simulink library "libFSArray"  (R2020a)
settings: Solver=VariableStepAuto  StartTime=0.0  StopTime=10.0  RelTol=1e-3
libraries: powerlib x2, $bdroot x1, re_lib x1
settings Model: Creator=pkoralew  LastModifiedBy=pkoralew

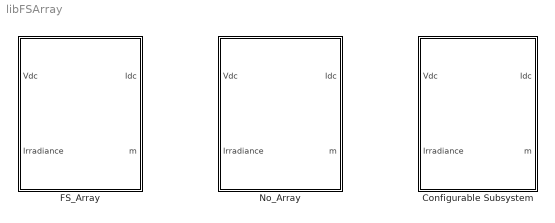
== system libFSArray ==
  Configurable Subsystem : Subsystem  BlockChoice=FS_Array
      settings: TemplateBlock=self  MemberBlocks=FS_Array,No_Array
  FS_Array : Subsystem
  No_Array : Subsystem

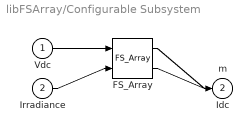
== system libFSArray/Configurable Subsystem ==
  Vdc : Inport
  Irradiance : Inport  Port=2
  FS_Array : $bdroot/FS_Array  SystemSampleTime=-1  Latency=0  AutoFrameSizeCalculation=off
  Idc : Outport
  m : Outport  Port=2
  wires:
  Vdc/1 -> FS_Array/1
  Irradiance/1 -> FS_Array/2
  FS_Array/1 -> Idc/1
  FS_Array/2 -> m/1

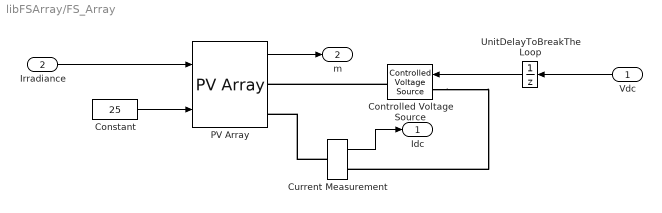
== system libFSArray/FS_Array ==
  Vdc : Inport
  Irradiance : Inport  Port=2
  Constant : Constant  Value=25
  Controlled Voltage Source : powerlib/Electrical Sources/Controlled Voltage Source  Initialize=on  Source_Type=AC  Amplitude=0  Phase=0  Frequency=0  Measurements=None
  Current Measurement : powerlib/Measurements/Current Measurement  PhasorSimulation=off  OutputType=Complex  PSBequivalent=0
  PV Array : re_lib/Solar/PV Array  Npar=300  Nser=18  PlotType=array @ 1000 W/m2 & specified temperatures  S_vec="[ 1000  500  100 ]"  Temp_C_vec="[ 45 25  ]"  ModuleName=First Solar FS-390  PlotWhenSelected=off  Pm=90.036  Ncell=77  Voc=61  Isc=2.04  Vm=49.2  Im=1.83  beta_Voc_pc=-0.236  alpha_Isc_pc=0.04299  beta_Voc=-0.14396  alpha_Isc=0.000877  IL=2.0554  I0=3.4814e-13  nI=1.0515  Rsh=377.2704  Rs=2.8667  RobustModel=off  RobustCellTemperature=25  BAL=on  Tc=1e-6  Tfilter=5e-5
  UnitDelayToBreakTheLoop : UnitDelay  InitialCondition=1000  SampleTime=-1  HasFrameUpgradeWarning=on
  Idc : Outport
  m : Outport  Port=2
  wires:
  Vdc/1 -> UnitDelayToBreakTheLoop/1
  PV Array/1 -> m/1
  UnitDelayToBreakTheLoop/1 -> Controlled Voltage Source/1
  Current Measurement/1 -> Idc/1
  Constant/1 -> PV Array/2
  Irradiance/1 -> PV Array/1
  connections:
  Controlled Voltage Source/RConn1 -- PV Array/RConn1
  Controlled Voltage Source/LConn1 -- Current Measurement/RConn1
  Current Measurement/LConn1 -- PV Array/RConn2

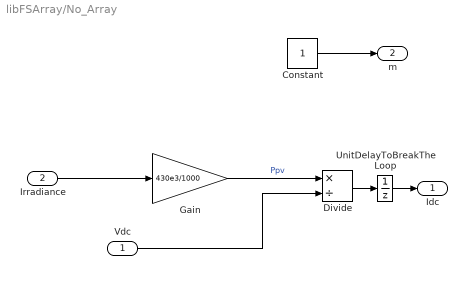
== system libFSArray/No_Array ==
  Vdc : Inport
  Irradiance : Inport  Port=2
  Constant : Constant
  Divide : Product  Inputs=*/
  Gain : Gain  Gain=430e3/1000
  UnitDelayToBreakTheLoop : UnitDelay  InitialCondition=1000  SampleTime=-1  HasFrameUpgradeWarning=on
  Idc : Outport
  m : Outport  Port=2
  wires:
  Constant/1 -> m/1
  Divide/1 -> UnitDelayToBreakTheLoop/1
  Irradiance/1 -> Gain/1
  Gain/1 -> Divide/1  "Ppv"
  Vdc/1 -> Divide/2
  UnitDelayToBreakTheLoop/1 -> Idc/1
